simulink model "pidmodel12"  (R2013a)
settings: Solver=ode45  StartTime=0.0  StopTime=100  RelTol=1e-1
values from neighbouring files (symbols this model uses):
  A = [0,0,1,0;0,0,0,1;-0,-12,-15,0;0,-3,-2,0]    [at.m]
  B = [0;0;-2;-3]    [at.m]
  C = [1,0,0,0;0,1,0,0;0,0,1,0;0,0,0,1]    [at.m]
  D = [0;0;0;0]    [at.m]
settings Model: Creator=user  LastModifiedBy=user
settings SolverCC: ZeroCrossAlgorithm=Adaptive

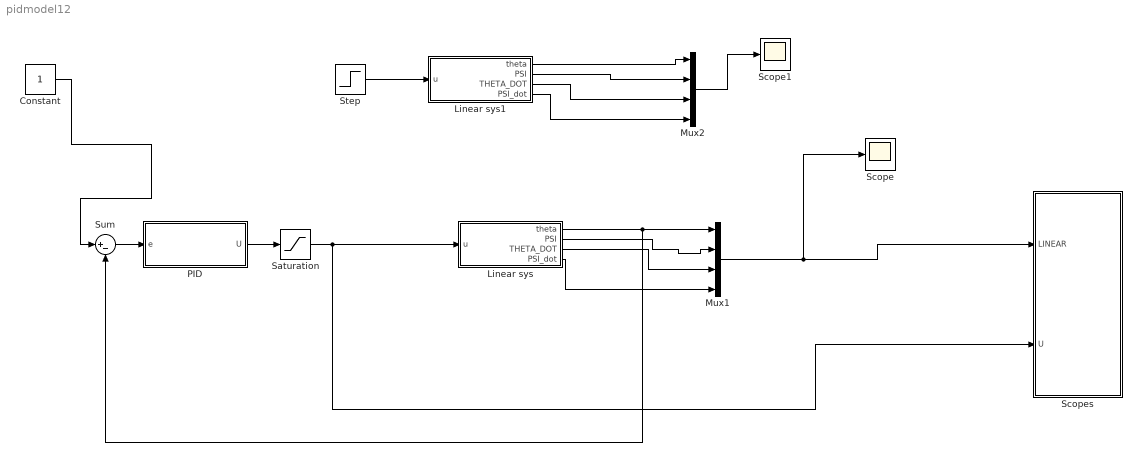
== system pidmodel12 ==
  Constant : Constant
  Linear sys : Subsystem
  Linear sys1 : Subsystem
  Mux1 : Mux
  Mux2 : Mux
  "PID " : Subsystem
  Saturation : Saturate  UpperLimit=1
  Scope : Scope
  Scope1 : Scope
      settings: SaveName=ScopeData2
  Scopes : Subsystem
  Step : Step  SampleTime=0
  Sum : Sum  Inputs=|+-
  wires:
  Sum/1 -> "PID "/1(e)
  "PID "/1(U) -> Saturation/1
  Linear sys/2(PSI) -> Mux1/2
  Linear sys/3(THETA_DOT) -> Mux1/3
  Mux1/1 -> Scope/1, Scopes/1(LINEAR)
  Saturation/1 -> Scopes/2(U), Linear sys/1(u)
  ? -> ?
  Linear sys/1(theta) -> Sum/2, Mux1/1
  Linear sys/4(PSI_dot) -> Mux1/4
  Constant/1 -> Sum/1
  Step/1 -> Linear sys1/1(u)
  Mux2/1 -> Scope1/1
  Linear sys1/1(theta) -> Mux2/1
  Linear sys1/2(PSI) -> Mux2/2
  Linear sys1/3(THETA_DOT) -> Mux2/3
  Linear sys1/4(PSI_dot) -> Mux2/4

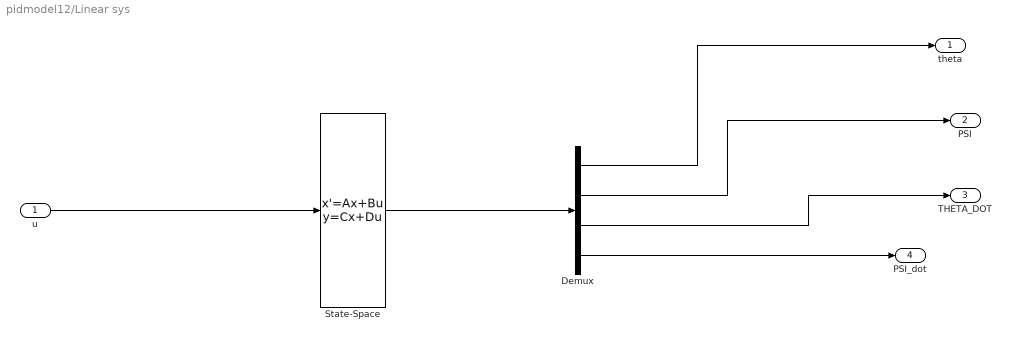
== system pidmodel12/Linear sys ==
  u : Inport
  Demux : Demux
  State-Space : StateSpace  A=A  B=B  C=C  D=D  X0=10
  theta : Outport
  PSI : Outport  Port=2
  THETA_DOT : Outport  Port=3
  PSI_dot : Outport  Port=4
  wires:
  u/1 -> State-Space/1
  State-Space/1 -> Demux/1
  Demux/1 -> theta/1
  Demux/2 -> PSI/1
  Demux/3 -> THETA_DOT/1
  Demux/4 -> PSI_dot/1

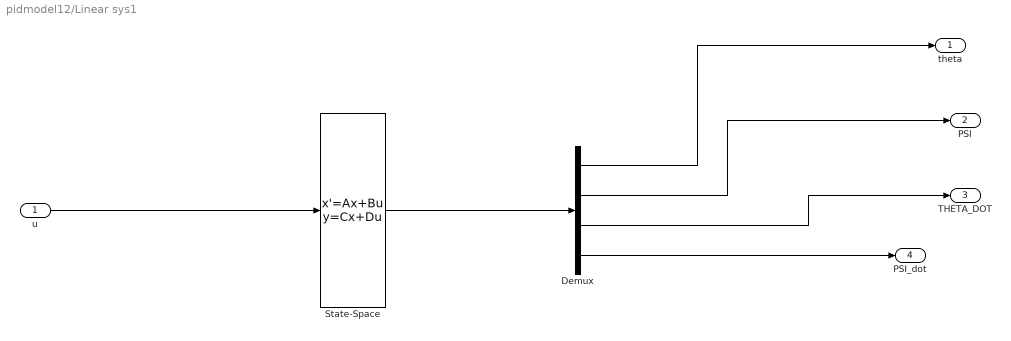
== system pidmodel12/Linear sys1 ==
  u : Inport
  Demux : Demux
  State-Space : StateSpace  A=A  B=B  C=C  D=D
  theta : Outport
  PSI : Outport  Port=2
  THETA_DOT : Outport  Port=3
  PSI_dot : Outport  Port=4
  wires:
  u/1 -> State-Space/1
  State-Space/1 -> Demux/1
  Demux/1 -> theta/1
  Demux/2 -> PSI/1
  Demux/3 -> THETA_DOT/1
  Demux/4 -> PSI_dot/1

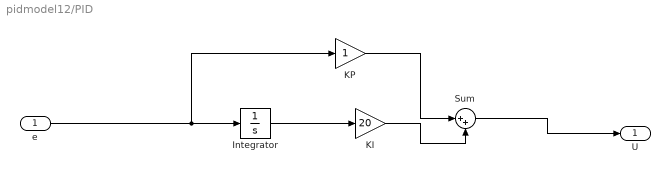
== system pidmodel12/PID  ==
  e : Inport
  Integrator : Integrator
  KI : Gain  Gain=20
  KP : Gain
  Sum : Sum  Inputs=|++
  U : Outport
  wires:
  e/1 -> KP/1, Integrator/1
  Integrator/1 -> KI/1
  Sum/1 -> U/1
  KP/1 -> Sum/1
  KI/1 -> Sum/2

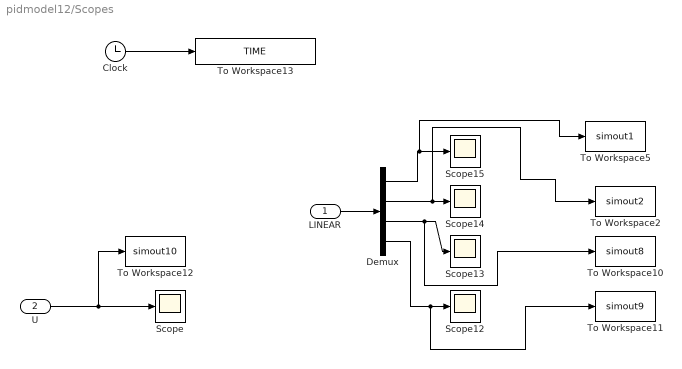
== system pidmodel12/Scopes ==
  LINEAR : Inport
  U : Inport  Port=2
  Clock : Clock
  Demux : Demux
  Scope{,12..15} (5 alike) : Scope
      Scope12 settings: SaveName=ScopeData12
      Scope13 settings: SaveName=ScopeData13
      Scope14 settings: SaveName=ScopeData14
      Scope15 settings: SaveName=ScopeData15
  To Workspace10 : ToWorkspace  VariableName=simout8  SampleTime=-1  SaveFormat=Timeseries
  To Workspace11 : ToWorkspace  VariableName=simout9  SampleTime=-1  SaveFormat=Timeseries
  To Workspace12 : ToWorkspace  VariableName=simout10  SampleTime=-1  SaveFormat=Timeseries
  To Workspace13 : ToWorkspace  VariableName=TIME  SampleTime=-1  SaveFormat=Timeseries
  To Workspace2 : ToWorkspace  VariableName=simout2  SampleTime=-1  SaveFormat=Timeseries
  To Workspace5 : ToWorkspace  VariableName=simout1  SampleTime=-1  SaveFormat=Timeseries
  wires:
  LINEAR/1 -> Demux/1
  Demux/1 -> To Workspace5/1, Scope15/1
  Demux/3 -> To Workspace10/1, Scope13/1
  Demux/2 -> To Workspace2/1, Scope14/1
  Demux/4 -> To Workspace11/1, Scope12/1
  U/1 -> To Workspace12/1, Scope/1
  Clock/1 -> To Workspace13/1
